simulink model "uwyp1f_1"  (Simulink 9.3)
settings: Solver=VariableStepAuto  StartTime=0.0  StopTime=0.1  FixedStep=1e-4  MaxStep=2e-3  RelTol=1e-3  EnableMultiTasking=on
libraries: powerlib x15, powerlib_extras x5, simulink x2
settings Model: LogicAnalyzerSignalOrdering=2aeaeec1-2b4b-4dbf-87fa-a87cff347230  Creator=Teacher  LastModifiedBy=ogure
settings SolverCC: SolverResetMethod=Robust  AutoInsertRateTranBlk=on
settings DataIOCC: SignalLoggingSaveFormat=Dataset  OutputSaveName=I1
settings OptimizationCC: InitFltsAndDblsToZero=on
settings DebuggingCC: SaveWithParameterizedLinksMsg=none  SignalResolutionControl=TryResolveAllWithWarning  SolverPrmCheckMsg=warning  MultiTaskDSMMsg=warning  MultiTaskCondExecSysMsg=none
settings GRTTargetCC: TargetFcnLib=ansi_tfl_tmw.mat  GeneratePreprocessorConditionals=Disable all
settings ConfigComp: CovSFcnEnable=off
settings SimscapeCC: SimscapeNormalizeSystem=off

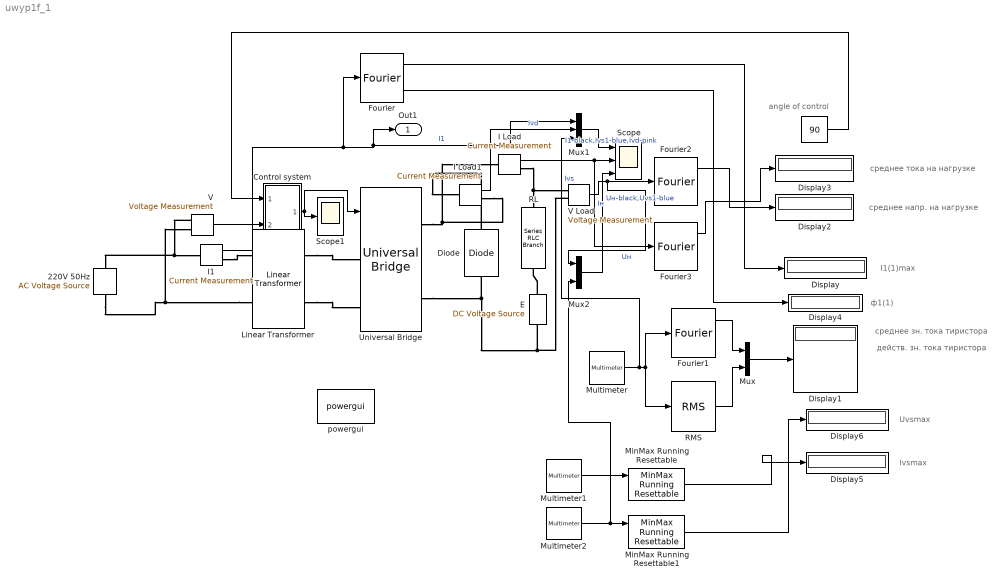
== system uwyp1f_1 ==
  note: действ. зн. тока тиристора
  note: среднее зн. тока тиристора
  note: среднее тока на нагрузке
  note: среднее напр. на нагрузке
  note: angle of control
  note: ф1(1)
  note: I1(1)max
  note: Ivsmax
  note: Uvsmax
  " " : Constant  Value=90
  220V 50Hz : powerlib/Electrical Sources/AC Voltage Source  Amplitude=310  Phase=0  Frequency=50  SampleTime=2*10^-4  Measurements=None  BusType=swing  Pref=10e3  Qref=0  Qmin=-inf  Qmax=+inf
      settings: SourceProductName=Simscape Electrical
  Control system : Subsystem
  Diode : powerlib/Power Electronics/Diode  Ron=0.1  Lon=0  Vf=0.8  IC=0  UseSnubber=off  Rs=1e6  Cs=1e-9  Measurements=off
      settings: SourceProductName=Simscape Electrical
  Display{,1..6} (7 alike) : Display
  E : powerlib/Electrical Sources/DC Voltage Source  Amplitude=75  Measurements=None
      settings: SourceProductName=Simscape Electrical
  Fourier : powerlib_extras/Measurements/Fourier  f1=50  n=1
      settings: SourceProductName=Simscape Electrical  SourceProductBaseCode=PS
  Fourier1 : powerlib_extras/Measurements/Fourier  f1=50  n=0
      settings: SourceProductName=Simscape Electrical  SourceProductBaseCode=PS
  Fourier2 : powerlib_extras/Measurements/Fourier  f1=50  n=0
      settings: SourceProductName=Simscape Electrical  SourceProductBaseCode=PS
  Fourier3 : powerlib_extras/Measurements/Fourier  f1=50  n=0
      settings: SourceProductName=Simscape Electrical  SourceProductBaseCode=PS
  I Load : powerlib/Measurements/Current Measurement  PhasorSimulation=off  OutputType=Complex  PSBequivalent=0
      settings: SourceProductName=Simscape Electrical
  I Load1 : powerlib/Measurements/Current Measurement  PhasorSimulation=off  OutputType=Complex  PSBequivalent=0
      settings: SourceProductName=Simscape Electrical
  I1 : powerlib/Measurements/Current Measurement  PhasorSimulation=off  OutputType=Complex  PSBequivalent=0
      settings: SourceProductName=Simscape Electrical
  Linear Transformer : powerlib/Elements/Linear Transformer  UNITS=pu  NominalPower=[ 20000 50 ]  winding1="[ 310/sqrt(2)  0.2  0.8 ]"  winding2="[ 560/sqrt(2) 0.2  0.8 ]"  ThreeWindings=off  winding3=[ 60e3 0.005 0.02 ]  RmLm=[ 500 500 ]  Measurements=None  DataType=off
      settings: SourceProductName=Simscape Electrical
  MinMax Running Resettable : simulink/Math Operations/MinMax Running Resettable  Function=max  vinit=0.0
  MinMax Running Resettable1 : simulink/Math Operations/MinMax Running Resettable  Function=min  vinit=0.0
  Multimeter : powerlib/Measurements/Multimeter  PhasorSimulation=off  OutputType=Complex  sel=7  L=10  Gain=1  yselected={'Isw1: Universal Bridge'};  PSBOutputType=1  PSBequivalent=0  AxesSetting=[0,0.1,-100,100]  Display=0  SavedBlockNames=-11
      settings: SourceProductName=Simscape Electrical
  Multimeter1 : powerlib/Measurements/Multimeter  PhasorSimulation=off  OutputType=Complex  sel=7  L=10  Gain=1  yselected={'Isw1: Universal Bridge'};  PSBOutputType=1  PSBequivalent=0  AxesSetting=[0,0.1,-100,100]  Display=0  SavedBlockNames=-11
      settings: SourceProductName=Simscape Electrical
  Multimeter2 : powerlib/Measurements/Multimeter  PhasorSimulation=off  OutputType=Complex  sel=1  L=10  Gain=1  yselected={'Usw1: Universal Bridge'};  PSBOutputType=1  PSBequivalent=0  AxesSetting=[0,0.1,-100,100]  Display=0  SavedBlockNames=-11
      settings: SourceProductName=Simscape Electrical
  Mux : Mux  Inputs=2
  Mux1 : Mux  Inputs=3
  Mux2 : Mux  Inputs=3
  RL : powerlib/Elements/Series RLC Branch  LConnTagsString=__new0  RConnTagsString=__new0  BranchType=RL  Resistance=90  Inductance=900/(2*pi*100)  SetiL0=off  InitialCurrent=0  Capacitance=inf  Setx0=off  InitialVoltage=0  Measurements=None
      settings: SourceProductName=Simscape Electrical
  RMS : powerlib_extras/Measurements/RMS  f1=50
      settings: SourceProductName=Simscape Electrical  SourceProductBaseCode=PS
  Scope : Scope  NumInputPorts=3
  Scope1 : Scope
  Universal Bridge : powerlib/Power Electronics/Universal Bridge  Arms=2  SnubberResistance=1e6  SnubberCapacitance=1e-9  Device=Thyristors  Ron=0.1  Lon=0  ForwardVoltages="[  0  0  ]"  ForwardVoltage=0.8  GTOparameters=[ 10e-6 , 20e-6 ]  IGBTparameters=[ 1e-6 , 2e-6 ]  Measurements=All voltages and currents  Measurements_2=None  converterType=Rectifier
      settings: SourceProductName=Simscape Electrical
  V : powerlib/Measurements/Voltage Measurement  PhasorSimulation=off  OutputType=Complex  PSBequivalent=0
      settings: SourceProductName=Simscape Electrical
  V Load : powerlib/Measurements/Voltage Measurement  PhasorSimulation=off  OutputType=Complex  PSBequivalent=0
      settings: SourceProductName=Simscape Electrical
  powergui : powerlib/powergui  Priority=1  SimulationMode=Continuous  SampleTime=2e-6  frequency=60  Iterations=50  frequencyindice=50  Pbase=100e6  ErrMax=1e-4  UnitsV=kV  UnitsW=MW  buscounter=0  FunctionMessages=off  echomessages=off  EnableUseOfTLC=off  CurrentSourceSwitches=off  DisableSnubberDevices=off  DisableRonSwitches=off  DisableVfSwitches=off  DisplayEquations=off  AutomaticDiscreteSolvers=off  SolverType=Tustin/Backward Euler (TBE)  Interpol=off  ExternalGateDelay=off  methode=off  Ts=100  x0status=blocks  SPID=off  SwTol=0  HookPort=off  NonlinearTolerance=0  nMaxIteration=15  ContinueOnMaxIteration=off  RestoreLinks=warning  ResistiveCurrentMeasurement=off  Frange=[0:2:500]  Ylog=off  Xlog=on  ShowGrid=off  save=off  variable=ZData  structure=0  ZoomFFT=off  StartTime=0.0  cycles=1  DisplayStyle=1  fundamental=60  FreqAxis=off  MaxFrequency=1000  frequencyindicesteady=1  RmsSteady=1  display=off
      settings: SourceProductName=Simscape Electrical
  Out1 : Outport
  wires:
  I1/1 -> Fourier/1, Mux1/1, Out1/1  "I1"
  I Load/1 -> Scope/2, Fourier3/1  "Iн"
  Fourier1/1 -> Mux/1
  Multimeter/1 -> Mux1/3, RMS/1, Fourier1/1  "Ivs"
  Mux/1 -> Display1/1
  RMS/1 -> Mux/2
  Fourier2/1 -> Display2/1
  Fourier3/1 -> Display3/1
  V Load/1 -> Mux2/1, Fourier2/1  "Uн"
  Control system/1(Out1) -> Scope1/1, Universal Bridge/1
  V/1 -> Control system/2(In2)
  " "/1 -> Control system/1(In1)
  Fourier/2 -> Display4/1
  Fourier/1 -> Display/1
  MinMax Running Resettable/1 -> Display5/1
  MinMax Running Resettable1/1 -> Display6/1
  Multimeter1/1 -> MinMax Running Resettable/1
  Multimeter2/1 -> Mux2/3, MinMax Running Resettable1/1
  Mux1/1 -> Scope/1  "I1-black,Ivs1-blue,Ivd-pink"
  Mux2/1 -> Scope/3  "Uн-black,Uvs1-blue"
  I Load1/1 -> Mux1/2  "Ivd"
  connections:
  V/LConn1 -- 220V 50Hz/RConn1 -- I1/LConn1
  Linear Transformer/LConn2 -- 220V 50Hz/LConn1 -- V/LConn2
  I1/RConn1 -- Linear Transformer/LConn1
  Linear Transformer/RConn1 -- Universal Bridge/LConn1
  Linear Transformer/RConn2 -- Universal Bridge/LConn2
  E/RConn1 -- RL/RConn1
  Universal Bridge/RConn2 -- V Load/LConn2 -- E/LConn1 -- Diode/LConn1
  Universal Bridge/RConn1 -- I Load/LConn1 -- I Load1/RConn1
  I Load/RConn1 -- RL/LConn1 -- V Load/LConn1
  Diode/RConn1 -- I Load1/LConn1

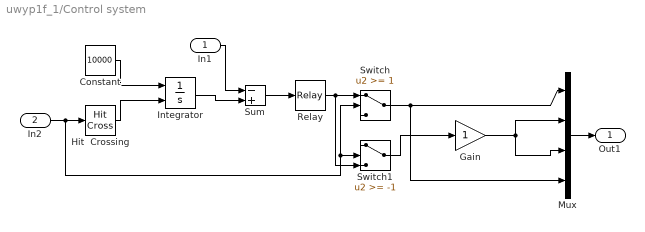
== system uwyp1f_1/Control system ==
  In1 : Inport
  In2 : Inport  Port=2
  Constant : Constant  Value=10000  VectorParams1D=off
  Gain : Gain
  Hit  Crossing : HitCross
  Integrator : Integrator  ExternalReset=rising
  Mux : Mux
  Relay : Relay  OnSwitchValue=0.1  OffSwitchValue=-0.1
  Sum : Sum  Inputs=-+
  Switch : Switch  Threshold=1
  Switch1 : Switch  Threshold=-1
  Out1 : Outport
  wires:
  In2/1 -> Switch/2, Switch1/2, Hit  Crossing/1
  Switch1/1 -> Gain/1
  Relay/1 -> Switch1/3, Switch/1
  Sum/1 -> Relay/1
  Integrator/1 -> Sum/2
  Hit  Crossing/1 -> Integrator/2
  Constant/1 -> Integrator/1
  Gain/1 -> Mux/3, Mux/2
  Switch/1 -> Mux/1, Mux/4
  In1/1 -> Sum/1
  Mux/1 -> Out1/1
